simulink model "Reas_Graph"  (R2025a)
settings: Solver=FixedStepAuto  StartTime=0.0  StopTime=inf  FixedStep=0.0005  RelTol=1e-3
undefined symbols (not defined in the file): Blocking, Non
libraries: amg_usbconverter_n_connect_lib x2, waijung_addon_module x1
settings Model: Creator=ACER  LastModifiedBy=ACER

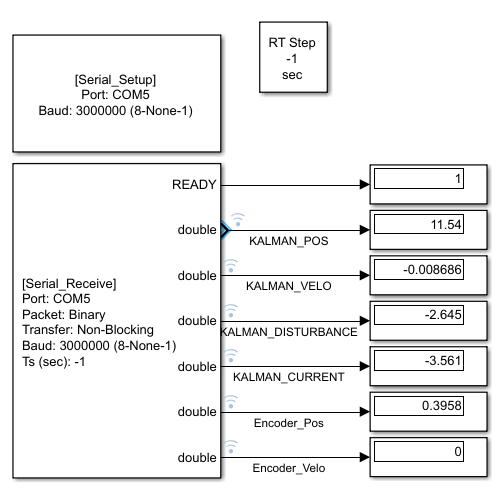
[thumbnail: Simulink's stored preview of the top-level diagram]
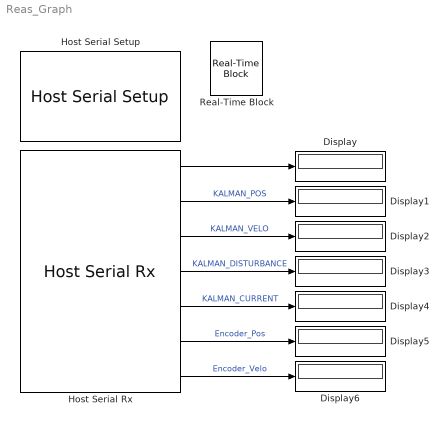
== system Reas_Graph ==
  Display{,1..6} (7 alike) : Display
  Host Serial Rx : amg_usbconverter_n_connect_lib/Host Serial Rx  conf=rx  port=<auto>  baudrate=3000000  databits=8  parity=None  stopbit=1  flowcontrol=None  transfer=Non-Blocking  timeout=5  packetmode=Binary  enableinitialvalues=off  initialvalues=[]  binheader='0x0f'  binterminator='0'  porttype_double=6  porttype_single=0  porttype_int8=0  porttype_uint8=0  porttype_int16=0  porttype_uint16=0  porttype_int32=0  porttype_uint32=0  asciiformat='%d,%f'  rx_asciiterminator="CRLF (0x0D 0x0A - \"\\r\\n\")"  tx_asciiterminator="CRLF (0x0D 0x0A - \"\\r\\n\")"  sampletime=-1  enablecustomportlabel=off  cinputportlabel=0  coutputportlabel=A  portpinstr=0  blockid=HostSerialRx  inputporttype=[]  inputportwidth=[]  inputportlabel={}  outputporttype=[3 0 0 0 0 0 0]  outputportwidth=[1 1 1 1 1 1 1]  outputportlabel={'READY','double','double','double','double','double','double'}  compat=0  optionstring=[]  autoport='COM5'
  Host Serial Setup : amg_usbconverter_n_connect_lib/Host Serial Setup  conf=setup  port=<auto>  baudrate=3000000  databits=8  parity=None  stopbit=1  flowcontrol=None  transfer=Blocking  timeout=2  packetmode=Binary  initialvalues=[]  binheader='7E 7E'  binterminator='03 03'  porttype_double=0  porttype_single=1  porttype_int8=0  porttype_uint8=0  porttype_int16=0  porttype_uint16=0  porttype_int32=0  porttype_uint32=2  asciiformat='%d %u %x'  rx_asciiterminator="CRLF (0x0D 0x0A - \"\\r\\n\")"  tx_asciiterminator="CRLF (0x0D 0x0A - \"\\r\\n\")"  sampletime=-1  enablecustomportlabel=off  cinputportlabel=0  coutputportlabel=A  portpinstr=0  blockid=HostSerialSetup  inputporttype=[]  inputportwidth=[]  inputportlabel={}  outputporttype=[]  outputportwidth=[]  outputportlabel={}  compat=0  optionstring=[]  autoport='COM5'
  Real-Time Block : waijung_addon_module/Real-Time Block  Priority=0  setting=Default  sampletime=-1
      settings: SourceProductName=Misc
  wires:
  Host Serial Rx/1 -> Display/1
  Host Serial Rx/2 -> Display1/1  "KALMAN_POS"
  Host Serial Rx/4 -> Display3/1  "KALMAN_DISTURBANCE"
  Host Serial Rx/3 -> Display2/1  "KALMAN_VELO"
  Host Serial Rx/7 -> Display6/1  "Encoder_Velo"
  Host Serial Rx/6 -> Display5/1  "Encoder_Pos"
  Host Serial Rx/5 -> Display4/1  "KALMAN_CURRENT"
